simulink model "saturation_block"  (R2020a)
settings: Solver=VariableStepAuto  StartTime=0.0  StopTime=10.0  RelTol=1e-3
libraries: simulink x6
settings Model: Creator=Ujwal  LastModifiedBy=Ujwal

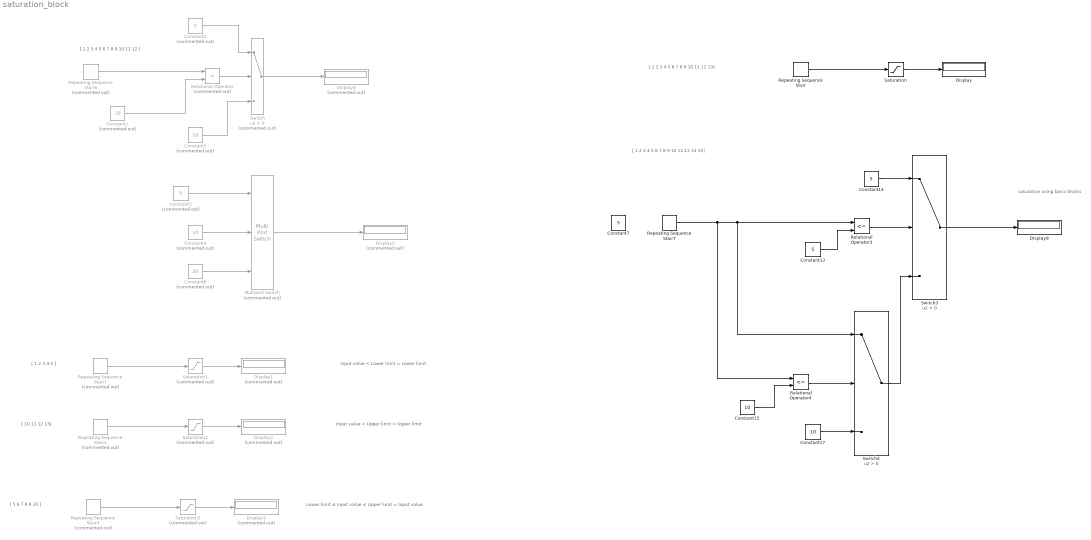
== system saturation_block ==
  note: saturation using basic blocks
  note: [ 1 2 3 4 5 6 7 8 9 10 12 13 14 15]
  note: [ 1 2 3 4 5 6 7 8 9 10 11 12 ]
  note: [ 5 6 7 8 9 10 ]
  note: [ 10 11 12 13]
  note: [ 1 2 3 4 5 ]
  note: Input value > Upper limit = Upper limit
  note: Input value < Lower limit = Lower limit
  note: Lower limit ≤ Input value ≤ Upper limit = Input value
  note: [ 1 2 3 4 5 6 7 8 9 10 11 12 13]
  Constant1 : Constant  Commented=on  Value=10
  Constant13 : Constant  Value=5
  Constant14 : Constant  Value=5
  Constant15 : Constant  Value=10
  Constant17 : Constant  Value=10
  Constant2 : Constant  Commented=on  Value=5
  Constant3 : Constant  Commented=on  Value=10
  Constant4 : Constant  Commented=on  Value=10
  Constant5 : Constant  Commented=on  Value=5
  Constant6 : Constant  Commented=on  Value=20
  Constant7 : Constant  Value=5
  Display : Display
  Display{1..5} (5 alike) : Display  Commented=on
  Display8 : Display
  Multiport Switch : MultiPortSwitch  Commented=on  DataPortOrder=Specify indices  DataPortIndices={10,20,}
  Relational Operator : RelationalOperator  Commented=on  Operator=<  OutDataTypeStr=boolean  RndMeth=Simplest
  Relational Operator3 : RelationalOperator  Operator=<=  OutDataTypeStr=boolean  RndMeth=Simplest
  Relational Operator4 : RelationalOperator  Operator=<=  OutDataTypeStr=boolean  RndMeth=Simplest
  Repeating Sequence Stair : simulink/Sources/Repeating Sequence Stair  OutValues=[ 1 2 3 4 5 6 7 8 9 10 11 12 13]  tsamp=-1  OutMin=[]  OutMax=[]  OutDataTypeStr=double  OutputDataTypeScalingMode=double  OutDataType=fixdt(0,8)  ConRadixGroup=Best Precision: Vector-wise  OutScaling=2^-12
  Repeating Sequence Stair1 : simulink/Sources/Repeating Sequence Stair  Commented=on  OutValues="[ 1 2 3 4 5 6 7 8 9 10 12 13  14 15]"  tsamp=-1  OutMin=[]  OutMax=[]  OutDataTypeStr=double  OutputDataTypeScalingMode=double  OutDataType=fixdt(0,8)  ConRadixGroup=Best Precision: Vector-wise  OutScaling=2^-12
  Repeating Sequence Stair2 : simulink/Sources/Repeating Sequence Stair  Commented=on  OutValues=[ 10 11 12 13]  tsamp=-1  OutMin=[]  OutMax=[]  OutDataTypeStr=double  OutputDataTypeScalingMode=double  OutDataType=fixdt(0,8)  ConRadixGroup=Best Precision: Vector-wise  OutScaling=2^-12
  Repeating Sequence Stair3 : simulink/Sources/Repeating Sequence Stair  Commented=on  OutValues="[  5 6 7 8 9 10 ]"  tsamp=-1  OutMin=[]  OutMax=[]  OutDataTypeStr=double  OutputDataTypeScalingMode=double  OutDataType=fixdt(0,8)  ConRadixGroup=Best Precision: Vector-wise  OutScaling=2^-12
  Repeating Sequence Stair6 : simulink/Sources/Repeating Sequence Stair  Commented=on  OutValues=[ 1 2 3 4 5 6 7 8 9 10 11 12 ]  tsamp=-1  OutMin=[]  OutMax=[]  OutDataTypeStr=double  OutputDataTypeScalingMode=double  OutDataType=fixdt(0,8)  ConRadixGroup=Best Precision: Vector-wise  OutScaling=2^-12
  Repeating Sequence Stair7 : simulink/Sources/Repeating Sequence Stair  OutValues="[ 1 2 3 4 5 6 7 8 9 10 12 13  14 15]"  tsamp=-1  OutMin=[]  OutMax=[]  OutDataTypeStr=double  OutputDataTypeScalingMode=double  OutDataType=fixdt(0,8)  ConRadixGroup=Best Precision: Vector-wise  OutScaling=2^-12
  Saturation : Saturate  UpperLimit=10  LowerLimit=5
  Saturation1 : Saturate  Commented=on  UpperLimit=10  LowerLimit=5
  Saturation2 : Saturate  Commented=on  UpperLimit=10  LowerLimit=5
  Saturation3 : Saturate  Commented=on  UpperLimit=10  LowerLimit=5
  Switch : Switch  Commented=on  Criteria=u2 > Threshold
  Switch3 : Switch  Criteria=u2 > Threshold
  Switch4 : Switch  Criteria=u2 > Threshold
  wires:
  Repeating Sequence Stair/1 -> Saturation/1
  Saturation/1 -> Display/1
  Repeating Sequence Stair1/1 -> Saturation1/1
  Saturation1/1 -> Display1/1
  Repeating Sequence Stair2/1 -> Saturation2/1
  Saturation2/1 -> Display2/1
  Repeating Sequence Stair3/1 -> Saturation3/1
  Saturation3/1 -> Display3/1
  Constant1/1 -> Relational Operator/2
  Relational Operator/1 -> Switch/2
  Constant2/1 -> Switch/1
  Constant3/1 -> Switch/3
  Switch/1 -> Display4/1
  Constant5/1 -> Multiport Switch/1
  Constant4/1 -> Multiport Switch/2
  Constant6/1 -> Multiport Switch/3
  Multiport Switch/1 -> Display5/1
  Repeating Sequence Stair6/1 -> Relational Operator/1
  Constant13/1 -> Relational Operator3/2
  Relational Operator3/1 -> Switch3/2
  Switch3/1 -> Display8/1
  Constant14/1 -> Switch3/1
  Repeating Sequence Stair7/1 -> Relational Operator3/1, Switch4/1, Relational Operator4/1
  Switch4/1 -> Switch3/3
  Relational Operator4/1 -> Switch4/2
  Constant15/1 -> Relational Operator4/2
  Constant17/1 -> Switch4/3
